simulink subsystem "D1_Kerek"  (R2024b)
settings: Solver=VariableStepAuto  StartTime=0.0  StopTime=10.0  RelTol=1e-3
values from neighbouring files (symbols this model uses):
  b = 5e-4    (= 0.0005)    [D1script.m]
  c = 0    [D1script.m]    (also in disp.mat; onlabscript.m)
  r = 0.05    [TestingScript.m]    (also in compare.m = Mod.Mod.signals(2).values; disp.mat)
settings Model: Creator=Asus  LastModifiedBy=Asus

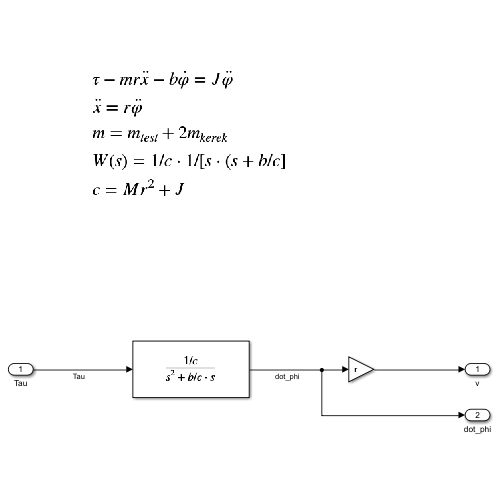
[thumbnail: Simulink's stored preview of the top-level diagram]
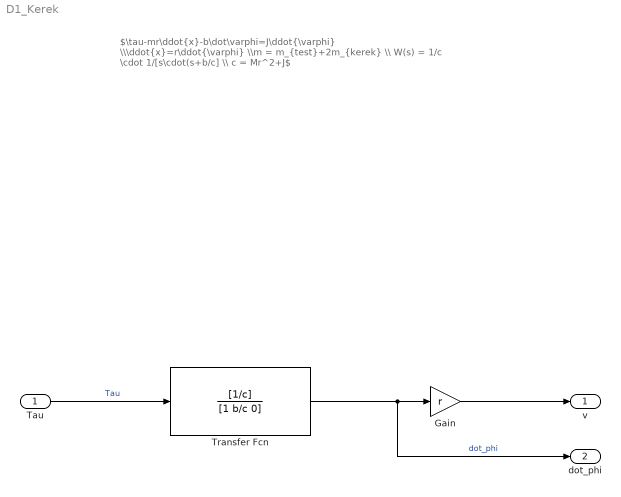
== system D1_Kerek ==
  note: $\tau-mr\ddot{x}-b\dot\varphi=J\ddot{\varphi} \\\ddot{x}=r\ddot{\varphi} \\m = m_{test}+2m_{kerek} \\ W(s) = 1/c \cdot 1/[s\cdot(s+b/c] \\ c = Mr^2+J$
  Tau : Inport
  Gain : Gain  Gain=r
  Transfer Fcn : TransferFcn  Numerator=[1/c]  Denominator=[1 b/c 0]
  v : Outport
  dot_phi : Outport  Port=2
  wires:
  Tau/1 -> Transfer Fcn/1  "Tau"
  Transfer Fcn/1 -> dot_phi/1, Gain/1  "dot_phi"
  Gain/1 -> v/1
